simulink library "nmc"  (R2015b)
settings: Solver=ode45  SolverMode=SingleTasking  StartTime=0.0  StopTime=10.0  RelTol=1e-3
undefined symbols (not defined in the file): AnkleStance, AnkleSwing, c, c_jointstop, CtrlPar_FP_List, CtrlPar_FP_R_List, CtrlPar_LL_List, CtrlPar_St_List, CtrlPar_St_R_List, CtrlPar_Sw_List, CtrlPar_Sw_R_List, CtrlPar_theta0_List, CtrlPar_Tr_List, CtrlPar_Tr_R_List, CtrlPar_VelocityFile_List, D1G_HAT, eref, FmaxBFSH, FmaxGAS, FmaxGLU, FmaxHAB, FmaxHAD, FmaxHAM, FmaxHFL, FmaxRF, FmaxSOL, FmaxTA, FmaxVAS, init_a_tgt, init_a_tgtR, K, leg_l, LongDelay, LongLoopDelay, loptBFSH, loptGAS, loptGLU, loptHAB, loptHAD, loptHAM, loptHFL, loptRF, loptSOL, loptTA, loptVAS, lslackBFSH, lslackGAS, lslackGLU, lslackHAB, lslackHAD, lslackHAM, lslackHFL, lslackRF, lslackSOL, lslackTA, lslackVAS, magnitude, maxLoad_control_List, MeanStepsAnkle, MidDelay ... (+99)
libraries: nmc x63, simulink x31, simulink_extras x30, LopesDevelopmentLibrary x3
(part 3 of 10)

== system nmc/LopesToGeyer_angles/AnklePredictorRight/LeftSwing ==
  MeasPhase : Inport
  Clock : Clock
      settings: Decimation=1E6
  Constant : Constant  Value=MeanStepsAnkle
  "Frequency " : Stateflow chart  TreatAsAtomicUnit=on
  "mean_freq " : Outport
  count : Outport  Port=2
  wires:
  "Frequency "/1(count) -> count/1
  "Frequency "/2(mean_freq) -> "mean_freq "/1
  Clock/1 -> "Frequency "/1(time_sig)
  MeasPhase/1 -> "Frequency "/2(InSig)
  Constant/1 -> "Frequency "/3(N)

== system nmc/LopesToGeyer_angles/AnklePredictorRight/MeanReady? ==
  Compare To Constant : simulink/Logic and Bit Operations/Compare To Constant  relop=>  const=MeanStepsAnkle  OutDataTypeStr=boolean
  Compare To Constant1 : simulink/Logic and Bit Operations/Compare To Constant  relop=>  const=MeanStepsAnkle  OutDataTypeStr=boolean
  Logical Operator : Logic  AllPortsSameDT=off  OutDataTypeStr=boolean
  "Ready " : Outport
  wires:
  [CountStanceR] -> Compare To Constant/1
  [CountSwingR] -> Compare To Constant1/1
  Logical Operator/1 -> "Ready "/1
  Compare To Constant1/1 -> Logical Operator/1
  Compare To Constant/1 -> Logical Operator/2

== system nmc/LopesToGeyer_angles/AnklePredictorRight/Shape estimator left ==
  Cur_phase : Inport
  mean_freq_swing : Inport  Port=2
  mean_freq_stance : Inport  Port=3
  Enable : EnablePort  StatesWhenEnabling=reset  ZeroCross=off
  Compare To Constant : simulink/Logic and Bit Operations/Compare To Constant  relop===  const=0  OutDataTypeStr=boolean
  Compare To Constant1 : simulink/Logic and Bit Operations/Compare To Constant  relop===  const=1  OutDataTypeStr=boolean
  Cur_phase1 : InportShadow
  Phase 1 : Subsystem
  Phase 2 : Subsystem
  Switch : Switch  Criteria=u2 ~= 0
  Shape : Outport  OutputWhenDisabled=reset  InitialOutput=0
  wires:
  mean_freq_stance/1 -> Phase 2/1(mean_freq)
  mean_freq_swing/1 -> Phase 1/1(mean_freq)
  Compare To Constant1/1 -> Phase 2/Enable
  Compare To Constant/1 -> Phase 1/Enable
  Cur_phase1/1 -> Switch/2
  Phase 1/1(Shape_output) -> Switch/3
  Phase 2/1(Shape_output) -> Switch/1
  Switch/1 -> Shape/1
  Cur_phase/1 -> Compare To Constant1/1, Compare To Constant/1

== system nmc/NMC Model/Global to Body frame/body pitch//roll//yaw in body frame --- x-axis: forward y-axis: leftward z-axis: parallel to gravity ==
  LHip : Inport
  dLHip : Inport  Port=2
  HAT : Inport  Port=3
  dHAT : Inport  Port=4
  RHip : Inport  Port=5
  dRHip : Inport  Port=6
  " Mean Hip Speed" : Gain  Gain=1/2
  "Dx, Dy" : Selector  InputPortWidth=3  IndexOptions=Index vector (dialog)  Indices=[1 2]  OutputSizes=1
  "Dx, Dz" : Selector  InputPortWidth=3  IndexOptions=Index vector (dialog)  Indices=[1 3]  OutputSizes=1
  "Dx, Dz1" : Selector  InputPortWidth=3  IndexOptions=Index vector (dialog)  Indices=[1 3]  OutputSizes=1
  "Dz, Dy" : Selector  InputPortWidth=3  IndexOptions=Index vector (dialog)  Indices=[3 2]  OutputSizes=1
  Mean Hip Position : Gain  Gain=1/2
  Mux1 : Mux  Inputs=2
  Mux2 : Mux  Inputs=2
  Mux3 : Mux  Inputs=2
  Sum1 : Sum
  Sum2 : Sum
  Sum4 : Sum  Inputs=-+
  Sum5 : Sum  Inputs=+-
  Theta : Fcn  Expr=atan2(u(1),u(2))
  Theta1 : Fcn  Expr=atan2(u(1),u(2))
  "dDx, dDy" : Selector  InputPortWidth=3  IndexOptions=Index vector (dialog)  Indices=[1 2]  OutputSizes=1
  "dDz, dDy" : Selector  InputPortWidth=3  IndexOptions=Index vector (dialog)  Indices=[3 2]  OutputSizes=1
  dTheta : Fcn  Expr=( u(2)*u(3) - u(1)*u(4) ) / D1G_HAT^2
  dTheta1 : Fcn  Expr=( u(2)*u(3) - u(1)*u(4) ) / D1G_HAT^2
  map1 : Subsystem
  map2 : Subsystem
  new_bases : Subsystem
  yaw1 : Fcn  Expr=atan2(-u(1)+u(3),-u(2)+u(4))
  th_pitch : Outport
  dth_pitch : Outport  Port=2
  th_roll : Outport  Port=3
  dth_roll : Outport  Port=4
  yaw : Outport  Port=5
  wires:
  yaw1/1 -> yaw/1
  Mux3/1 -> yaw1/1
  "Dx, Dz1"/1 -> Mux3/2
  "Dx, Dz"/1 -> Mux3/1
  dTheta1/1 -> dth_roll/1
  Theta1/1 -> th_roll/1
  "Dz, Dy"/1 -> Theta1/1, Mux1/1
  Mux1/1 -> dTheta1/1
  "dDz, dDy"/1 -> Mux1/2
  map2/1(v_new) -> "dDz, dDy"/1, "dDx, dDy"/1
  Sum5/1 -> map2/1(v)
  new_bases/1(bases) -> map2/2(basis), map1/2(basis)
  map1/1(v_new) -> "Dz, Dy"/1, "Dx, Dy"/1
  Sum4/1 -> map1/1(v)
  dTheta/1 -> dth_pitch/1
  Theta/1 -> th_pitch/1
  dRHip/1 -> Sum2/2
  dLHip/1 -> Sum2/1
  RHip/1 -> "Dx, Dz1"/1, new_bases/2(R), Sum1/2
  LHip/1 -> "Dx, Dz"/1, new_bases/1(L), Sum1/1
  "Dx, Dy"/1 -> Theta/1, Mux2/1
  " Mean Hip Speed"/1 -> Sum5/2
  Mean Hip Position/1 -> Sum4/1
  HAT/1 -> Sum4/2
  Sum2/1 -> " Mean Hip Speed"/1
  Sum1/1 -> Mean Hip Position/1
  Mux2/1 -> dTheta/1
  "dDx, dDy"/1 -> Mux2/2
  dHAT/1 -> Sum5/1

== system nmc/NMC Model/Global to Body frame/lateral d, v in body frame (left) ==
  body yaw : Inport
  d0 : Inport  Port=2
  dist : Inport  Port=3
  vel : Inport  Port=4
  Mux1 : Mux  Inputs=2
  Mux2 : Mux  Inputs=2
  Mux3 : Mux  Inputs=2
  Sum : Sum  Inputs=-+|
  body frame in transverse plane (xz-plane)1 : Fcn  Expr=u(2)*sin(u(1)) + u(3)*cos(u(1))
  body frame in transverse plane (xz-plane)2 : Fcn  Expr=u(2)*sin(u(1)) + u(3)*cos(u(1))
  "d, v" : Outport
  wires:
  Mux3/1 -> "d, v"/1
  body frame in transverse plane (xz-plane)1/1 -> Mux3/1
  vel/1 -> Mux2/2
  body frame in transverse plane (xz-plane)2/1 -> Mux3/2
  dist/1 -> Sum/2
  d0/1 -> Sum/1
  Mux2/1 -> body frame in transverse plane (xz-plane)2/1
  body yaw/1 -> Mux1/1, Mux2/1
  Mux1/1 -> body frame in transverse plane (xz-plane)1/1
  Sum/1 -> Mux1/2

== system nmc/NMC Model/Global to Body frame/lateral d, v in body frame (right) ==
  body yaw : Inport
  d0 : Inport  Port=2
  dist : Inport  Port=3
  vel : Inport  Port=4
  Mux1 : Mux  Inputs=2
  Mux2 : Mux  Inputs=2
  Mux3 : Mux  Inputs=2
  Sum : Sum  Inputs=-+|
  body frame in transverse plane (xz-plane)1 : Fcn  Expr=u(2)*sin(u(1)) + u(3)*cos(u(1))
  body frame in transverse plane (xz-plane)2 : Fcn  Expr=u(2)*sin(u(1)) + u(3)*cos(u(1))
  "d, v" : Outport
  wires:
  Mux3/1 -> "d, v"/1
  body frame in transverse plane (xz-plane)1/1 -> Mux3/1
  vel/1 -> Mux2/2
  body frame in transverse plane (xz-plane)2/1 -> Mux3/2
  dist/1 -> Sum/2
  d0/1 -> Sum/1
  Mux2/1 -> body frame in transverse plane (xz-plane)2/1
  body yaw/1 -> Mux1/1, Mux2/1
  Mux1/1 -> body frame in transverse plane (xz-plane)1/1
  Sum/1 -> Mux1/2

== system nmc/NMC Model/Global to Body frame/sagittal d, v in body frame (left) ==
  body yaw : Inport
  d0 : Inport  Port=2
  dist : Inport  Port=3
  vel : Inport  Port=4
  Mux1 : Mux  Inputs=2
  Mux2 : Mux  Inputs=2
  Mux3 : Mux  Inputs=2
  Sum : Sum  Inputs=-+|
  body frame in transverse plane (xz-plane)1 : Fcn  Expr=u(2)*cos(u(1)) - u(3)*sin(u(1))
  body frame in transverse plane (xz-plane)2 : Fcn  Expr=u(2)*cos(u(1)) - u(3)*sin(u(1))
  "d, v" : Outport
  wires:
  Mux3/1 -> "d, v"/1
  body frame in transverse plane (xz-plane)1/1 -> Mux3/1
  vel/1 -> Mux2/2
  body frame in transverse plane (xz-plane)2/1 -> Mux3/2
  dist/1 -> Sum/2
  d0/1 -> Sum/1
  Mux2/1 -> body frame in transverse plane (xz-plane)2/1
  body yaw/1 -> Mux1/1, Mux2/1
  Mux1/1 -> body frame in transverse plane (xz-plane)1/1
  Sum/1 -> Mux1/2

== system nmc/NMC Model/Global to Body frame/sagittal d, v in body frame (right) ==
  body yaw : Inport
  d0 : Inport  Port=2
  dist : Inport  Port=3
  vel : Inport  Port=4
  Mux1 : Mux  Inputs=2
  Mux2 : Mux  Inputs=2
  Mux3 : Mux  Inputs=2
  Sum : Sum  Inputs=-+|
  body frame in transverse plane (xz-plane)1 : Fcn  Expr=u(2)*cos(u(1)) - u(3)*sin(u(1))
  body frame in transverse plane (xz-plane)2 : Fcn  Expr=u(2)*cos(u(1)) - u(3)*sin(u(1))
  "d, v" : Outport
  wires:
  Mux3/1 -> "d, v"/1
  body frame in transverse plane (xz-plane)1/1 -> Mux3/1
  vel/1 -> Mux2/2
  body frame in transverse plane (xz-plane)2/1 -> Mux3/2
  dist/1 -> Sum/2
  d0/1 -> Sum/1
  Mux2/1 -> body frame in transverse plane (xz-plane)2/1
  body yaw/1 -> Mux1/1, Mux2/1
  Mux1/1 -> body frame in transverse plane (xz-plane)1/1
  Sum/1 -> Mux1/2

== system nmc/NMC Model/Higher Control Layer (Supra Spinal Control)/Double Support ==
  LStance : Inport
  RStance : Inport  Port=2
  Lalpha_tgt : Inport  Port=3
  Lphi34 : Inport  Port=4
  Lphi23 : Inport  Port=5
  LHip_tgt : Inport  Port=6
  Lphi34R : Inport  Port=7
  Ralpha_tgt : Inport  Port=8
  Rphi34 : Inport  Port=9
  Rphi23 : Inport  Port=10
  RHip_tgt : Inport  Port=11
  Rphi34R : Inport  Port=12
  Abs{,1..3} (4 alike) : Abs  ZeroCross=off
  Lalpha' : Fcn  Expr=u(1) - u(2)/2
  Logical Operator1 : Logic  Operator=NOR  AllPortsSameDT=off  OutDataTypeStr=boolean
  Logical Operator2 : Logic  Operator=NOT  AllPortsSameDT=off
  Logical Operator3 : Logic  AllPortsSameDT=off
  Logical Operator4 : Logic  AllPortsSameDT=off
  Logical Operator5 : Logic  AllPortsSameDT=off
  Mux1 : Mux  Inputs=2
  Mux5 : Mux  Inputs=2
  Ralpha' : Fcn  Expr=u(1) - u(2)/2
  Relational Operator : RelationalOperator  Operator=>  ZeroCross=off
  Sum{1,3,5,7} (4 alike) : Sum  Inputs=-+|
  Sum2 : Sum  Inputs=++|
  Sum4 : Sum  Inputs=++|
  RonL : Outport
  Flight : Outport  Port=2
  LonR : Outport  Port=3
  wires:
  Logical Operator3/1 -> Logical Operator4/1, Logical Operator5/1
  Relational Operator/1 -> Logical Operator4/2, Logical Operator2/1
  Logical Operator5/1 -> LonR/1
  Logical Operator2/1 -> Logical Operator5/2
  Logical Operator4/1 -> RonL/1
  Sum4/1 -> Relational Operator/2
  Abs3/1 -> Sum4/1
  Abs/1 -> Sum4/2
  Sum3/1 -> Abs3/1
  Rphi34R/1 -> Sum3/2
  RHip_tgt/1 -> Sum3/1
  Sum2/1 -> Relational Operator/1
  Abs1/1 -> Sum2/2
  Abs2/1 -> Sum2/1
  Sum1/1 -> Abs2/1
  Lphi34R/1 -> Sum1/2
  LHip_tgt/1 -> Sum1/1
  Logical Operator1/1 -> Flight/1
  Rphi23/1 -> Mux1/2
  Rphi34/1 -> Mux1/1
  Ralpha_tgt/1 -> Sum5/1
  Lphi23/1 -> Mux5/2
  Lphi34/1 -> Mux5/1
  Lalpha_tgt/1 -> Sum7/1
  RStance/1 -> Logical Operator1/2, Logical Operator3/2
  LStance/1 -> Logical Operator1/1, Logical Operator3/1
  Sum7/1 -> Abs1/1
  Sum5/1 -> Abs/1
  Mux1/1 -> Ralpha'/1
  Ralpha'/1 -> Sum5/2
  Mux5/1 -> Lalpha'/1
  Lalpha'/1 -> Sum7/2  "Lalpha"

== system nmc/NMC Model/Higher Control Layer (Supra Spinal Control)/SpeedCheck ==
  Abs : Abs
  Abs1 : Abs
  Compare To Constant : simulink/Logic and Bit Operations/Compare To Constant  relop===  const=0  OutDataTypeStr=boolean
  Logical Operator : Logic  Operator=OR  Inputs=3  AllPortsSameDT=off  OutDataTypeStr=boolean
  Relational Operator : RelationalOperator  Operator=>  OutDataTypeStr=boolean
  Relational Operator1 : RelationalOperator  Operator=>  OutDataTypeStr=boolean
  Select_front_v : Selector  InputPortWidth=2  IndexOptions=Index vector (dialog)  Indices=[2]  OutputSizes=1
  Select_side_v : Selector  InputPortWidth=2  IndexOptions=Index vector (dialog)  Indices=[2]  OutputSizes=1
  StandingStill : Constant  Value=0
  Switch : Switch  Criteria=u2 > Threshold
  "Walking " : Constant
  WalkOrStop : Outport
  wires:
  Logical Operator/1 -> Switch/2
  [StandingStillLimitFront] -> Relational Operator/2
  StandingStill/1 -> Switch/3
  [EnableStandingStill] -> Compare To Constant/1
  Relational Operator1/1 -> Logical Operator/3
  Relational Operator/1 -> Logical Operator/2
  Switch/1 -> WalkOrStop/1
  Abs1/1 -> Relational Operator1/1
  Select_side_v/1 -> Abs1/1
  Compare To Constant/1 -> Logical Operator/1
  [side_dv_L] -> Select_side_v/1
  Abs/1 -> Relational Operator/1
  Select_front_v/1 -> Abs/1
  [front_dv_L] -> Select_front_v/1
  "Walking "/1 -> Switch/1
  [StandingStillLimitSide] -> Relational Operator1/2

== system nmc/NMC Model/Muscle Actuation Layer/L Ankle Joint Limits ==
  note: Ankle Joint Limits
  phi [rad] : Inport
  dphi [rad/s] : Inport  Port=2
  Gain1 : Gain  Gain=c_jointstop
  Gain2 : Gain  Gain=-1
  Gain3 : Gain  Gain=c_jointstop
  Gain4 : Gain  Gain=1/w_max_jointstop
  Mux1 : Mux  Inputs=2
  Mux3 : Mux  Inputs=2
  Overextension Torque : Fcn  Expr="- u(1)  *  (1-u(2)) * (u(2)<1) * (u(1)>0)"
  Overflexion Torque : Fcn  Expr="- u(1)  *  (1-u(2)) * (u(2)<1) * (u(1)<0)"
  Sum : Sum  Inputs=|+-
  Sum1 : Sum  Inputs=|+-
  Sum2 : Sum
  overextension angle : Constant  Value=phi12_UpLimit
  overflexion angle : Constant  Value=phi12_LowLimit
  M_stop [Nm] : Outport
  wires:
  Overextension Torque/1 -> Sum2/1
  Overflexion Torque/1 -> Sum2/2
  Gain2/1 -> Mux3/2
  Sum2/1 -> M_stop [Nm]/1
  Mux1/1 -> Overflexion Torque/1
  overflexion angle/1 -> Sum1/2
  Sum1/1 -> Gain1/1
  Gain1/1 -> Mux1/1
  Gain4/1 -> Mux1/2, Gain2/1
  Sum/1 -> Gain3/1
  phi [rad]/1 -> Sum1/1, Sum/1
  overextension angle/1 -> Sum/2
  dphi [rad/s]/1 -> Gain4/1
  Gain3/1 -> Mux3/1
  Mux3/1 -> Overextension Torque/1

== system nmc/NMC Model/Muscle Actuation Layer/L BFSH ==
  note: Excitation Contraction Coupling
  note: BFSH Muscle-Tendon Dynamics
  STIM : Inport
  lmtc [m] : Inport  Port=2
  1 : Product  Inputs=**  SaturateOnIntegerOverflow=on  InputSameDT=on  OutDataTypeStr=Inherit: Same as first input
  1/lslack : Gain  Gain=1/lslackBFSH  SaturateOnIntegerOverflow=on  OutDataTypeStr=Inherit: Same as input  ParamDataTypeStr=Inherit: Same as input
  BE force-length relation : Subsystem
  CE force-length relation : Subsystem
  CE inverse force-velocity relation : Subsystem
  Constant : Constant  Value=lslackBFSH
  ECC TransferFcn : simulink_extras/Additional Linear/Transfer Fcn (with initial outputs)  N=[1]  D="[tau  1]"  Y0=preA  U0=0
      settings: AttributesFormatString=pre-activation: %<Y0>
  Fmax : Gain  Gain=FmaxBFSH  SaturateOnIntegerOverflow=on  OutDataTypeStr=Inherit: Same as input  ParamDataTypeStr=Inherit: Same as input
  Fv = Fse / (A*Fce) : Product  Inputs=*/  SaturateOnIntegerOverflow=on  InputSameDT=on  OutDataTypeStr=Inherit: Same as first input
  Integrator : Integrator  InitialConditionSource=external  LowerSaturationLimit=0.05  ZeroCross=off
  PE force-length relation : Subsystem
  SE force-length relation : Subsystem
  Sum : Sum  Inputs=|+-  SaturateOnIntegerOverflow=on  InputSameDT=on  OutDataTypeStr=Inherit: Same as first input
  Sum2 : Sum  Inputs=|-+  SaturateOnIntegerOverflow=on  InputSameDT=on  OutDataTypeStr=Inherit: Same as first input
  Sum3 : Sum  SaturateOnIntegerOverflow=on  InputSameDT=on  OutDataTypeStr=Inherit: Same as first input
  Sum4 : Sum  SaturateOnIntegerOverflow=on  InputSameDT=on  OutDataTypeStr=Inherit: Same as first input
  lce/lopt : Gain  Gain=1/loptBFSH  SaturateOnIntegerOverflow=on  OutDataTypeStr=Inherit: Same as input  ParamDataTypeStr=Inherit: Same as input
  vmax*lopt : Gain  Gain=vmaxBFSH*loptBFSH  SaturateOnIntegerOverflow=on  OutDataTypeStr=Inherit: Same as input  ParamDataTypeStr=Inherit: Same as input
  Fmtc : Outport  InitialOutput=0
  Lce : Outport  Port=2  InitialOutput=0
  Vce : Outport  Port=3  InitialOutput=0
  A : Outport  Port=4  InitialOutput=0
  wires:
  ECC TransferFcn/1 -> 1/2, A/1
  STIM/1 -> ECC TransferFcn/1
  CE inverse force-velocity relation/1(v[vmax]) -> vmax*lopt/1
  Sum3/1 -> Fv = Fse / (A*Fce)/2
  BE force-length relation/1(fbe [Fmax]) -> Sum4/2
  1/1 -> Sum3/2
  PE force-length relation/1(fpe [Fmax]) -> Sum3/1
  Sum4/1 -> Fv = Fse / (A*Fce)/1
  CE force-length relation/1(fce [Fmax]) -> 1/1
  Constant/1 -> Sum2/1
  Sum2/1 -> Integrator/2
  SE force-length relation/1(fse [Fmax]) -> Sum4/1, Fmax/1
  1/lslack/1 -> SE force-length relation/1(lse [lslack])
  Fmax/1 -> Fmtc/1  "Fmtc"
  lmtc [m]/1 -> Sum/1, Sum2/2  "lmtc"
  vmax*lopt/1 -> Vce/1, Integrator/1  "vce"
  Fv = Fse / (A*Fce)/1 -> CE inverse force-velocity relation/1(Fv[Fmax])  "fv"
  lce/lopt/1 -> PE force-length relation/1(lce [lopt]), BE force-length relation/1(lce [lopt]), CE force-length relation/1(lce [lopt])
  Sum/1 -> 1/lslack/1  "lse"
  Integrator/1 -> Lce/1, lce/lopt/1, Sum/2  "lce"

== system nmc/NMC Model/Muscle Actuation Layer/L BFSH Link ==
  note: BFSH Attachment
  phi23 [rad] : Inport
  Constant : Constant  Value=lslackBFSH+loptBFSH
  Constant1 : Constant  Value=rBFSH
  Constant2 : Constant  Value=phirefBFSH
  Gain4 : Gain  Gain=rhoBFSH
  Product : Product  RndMeth=Zero
  Sum2 : Sum  Inputs=|+-
  Sum5 : Sum  Inputs=|++
  lmtu [m] : Outport
  lever [m] : Outport  Port=2
  wires:
  Constant1/1 -> lever [m]/1, Product/2
  Sum2/1 -> Product/1
  Constant2/1 -> Sum2/2
  phi23 [rad]/1 -> Sum2/1
  Product/1 -> Gain4/1
  Gain4/1 -> Sum5/2
  Sum5/1 -> lmtu [m]/1
  Constant/1 -> Sum5/1

== system nmc/NMC Model/Muscle Actuation Layer/L GAS ==
  note: Excitation Contraction Coupling
  note: GAS Muscle-Tendon Dynamics
  STIM : Inport
  lmtc [m] : Inport  Port=2
  1 : Product  Inputs=**  SaturateOnIntegerOverflow=on  InputSameDT=on  OutDataTypeStr=Inherit: Same as first input
  1/lslack : Gain  Gain=1/lslackGAS  SaturateOnIntegerOverflow=on  OutDataTypeStr=Inherit: Same as input  ParamDataTypeStr=Inherit: Same as input
  BE force-length relation : Subsystem
  CE force-length relation : Subsystem
  CE inverse force-velocity relation : Subsystem
  Constant : Constant  Value=lslackGAS
  ECC TransferFcn : simulink_extras/Additional Linear/Transfer Fcn (with initial outputs)  N=[1]  D="[tau  1]"  Y0=preA  U0=0
      settings: AttributesFormatString=pre-activation: %<Y0>
  Fmax : Gain  Gain=FmaxGAS  SaturateOnIntegerOverflow=on  OutDataTypeStr=Inherit: Same as input  ParamDataTypeStr=Inherit: Same as input
  Fv = Fse / (A*Fce) : Product  Inputs=*/  SaturateOnIntegerOverflow=on  InputSameDT=on  OutDataTypeStr=Inherit: Same as first input
  Integrator : Integrator  InitialConditionSource=external  LowerSaturationLimit=0.05  ZeroCross=off
  PE force-length relation : Subsystem
  SE force-length relation : Subsystem
  Sum : Sum  Inputs=|+-  SaturateOnIntegerOverflow=on  InputSameDT=on  OutDataTypeStr=Inherit: Same as first input
  Sum2 : Sum  Inputs=|-+  SaturateOnIntegerOverflow=on  InputSameDT=on  OutDataTypeStr=Inherit: Same as first input
  Sum3 : Sum  SaturateOnIntegerOverflow=on  InputSameDT=on  OutDataTypeStr=Inherit: Same as first input
  Sum4 : Sum  SaturateOnIntegerOverflow=on  InputSameDT=on  OutDataTypeStr=Inherit: Same as first input
  lce/lopt : Gain  Gain=1/loptGAS  SaturateOnIntegerOverflow=on  OutDataTypeStr=Inherit: Same as input  ParamDataTypeStr=Inherit: Same as input
  vmax*lopt : Gain  Gain=vmaxGAS*loptGAS  SaturateOnIntegerOverflow=on  OutDataTypeStr=Inherit: Same as input  ParamDataTypeStr=Inherit: Same as input
  Fmtc : Outport  InitialOutput=0
  Lce : Outport  Port=2  InitialOutput=0
  Vce : Outport  Port=3  InitialOutput=0
  A : Outport  Port=4  InitialOutput=0
  wires:
  ECC TransferFcn/1 -> 1/2, A/1
  STIM/1 -> ECC TransferFcn/1
  CE inverse force-velocity relation/1(v[vmax]) -> vmax*lopt/1
  Sum3/1 -> Fv = Fse / (A*Fce)/2
  BE force-length relation/1(fbe [Fmax]) -> Sum4/2
  1/1 -> Sum3/2
  PE force-length relation/1(fpe [Fmax]) -> Sum3/1
  Sum4/1 -> Fv = Fse / (A*Fce)/1
  CE force-length relation/1(fce [Fmax]) -> 1/1
  Constant/1 -> Sum2/1
  Sum2/1 -> Integrator/2
  SE force-length relation/1(fse [Fmax]) -> Sum4/1, Fmax/1
  1/lslack/1 -> SE force-length relation/1(lse [lslack])
  Fmax/1 -> Fmtc/1  "Fmtc"
  lmtc [m]/1 -> Sum/1, Sum2/2  "lmtc"
  vmax*lopt/1 -> Vce/1, Integrator/1  "vce"
  Fv = Fse / (A*Fce)/1 -> CE inverse force-velocity relation/1(Fv[Fmax])  "fv"
  lce/lopt/1 -> PE force-length relation/1(lce [lopt]), BE force-length relation/1(lce [lopt]), CE force-length relation/1(lce [lopt])
  Sum/1 -> 1/lslack/1  "lse"
  Integrator/1 -> Lce/1, lce/lopt/1, Sum/2  "lce"

== system nmc/NMC Model/Muscle Actuation Layer/L GAS Link ==
  note: GAS Attachment
  phi23 [rad] : Inport
  phi12 [rad] : Inport  Port=2
  Constant1 : Constant  Value=phimaxGASk
  Constant2 : Constant  Value=phirefGASk
  Constant3 : Constant  Value=phimaxGASa
  Constant4 : Constant  Value=lslackGAS+loptGAS
  Constant5 : Constant  Value=phirefGASa
  Demux : Demux  Outputs=2
  Demux1 : Demux  Outputs=2
  Gain1 : Gain  Gain=rGASkmax
  Gain2 : Gain  Gain=rGASamax
  Gain3 : Gain  Gain=phiScaleGASa
  Gain5 : Gain  Gain=phiScaleGASk
  Gain6 : Gain  Gain=phiScaleGASk
  Gain7 : Gain  Gain=rhoGASk/phiScaleGASk
  Gain8 : Gain  Gain=phiScaleGASa
  Gain9 : Gain  Gain=rhoGASa/phiScaleGASa
  Mux : Mux  Inputs=2
  Mux1 : Mux  Inputs=2
  Sum1 : Sum  Inputs=-+
  Sum2 : Sum  Inputs=|+-
  Sum3 : Sum  Inputs=-+|
  Sum4 : Sum  Inputs=-+
  Sum5 : Sum  Inputs=++-
  Sum6 : Sum  Inputs=|+-
  Sum7 : Sum  Inputs=-+|
  length change term : Trigonometry
  length change term1 : Trigonometry
  offset correction term : Trigonometry
  offset correction term1 : Trigonometry
  variable lever term : Trigonometry  Operator=cos
  variable lever term1 : Trigonometry  Operator=cos
  lmtu [m] : Outport
  lever23 [m] : Outport  Port=2
  lever12 [m] : Outport  Port=3
  wires:
  Gain8/1 -> offset correction term1/1
  Gain3/1 -> length change term1/1, variable lever term1/1
  Gain2/1 -> Demux1/1
  Mux1/1 -> Gain2/1
  variable lever term1/1 -> Mux1/2
  Sum4/1 -> Mux1/1
  offset correction term1/1 -> Sum4/1
  length change term1/1 -> Sum4/2
  Constant5/1 -> Sum6/1
  Sum6/1 -> Gain8/1
  Constant3/1 -> Sum6/2, Sum7/1
  Sum7/1 -> Gain3/1
  phi12 [rad]/1 -> Sum7/2
  Gain6/1 -> offset correction term/1
  Gain5/1 -> length change term/1, variable lever term/1
  Gain1/1 -> Demux/1
  Mux/1 -> Gain1/1
  variable lever term/1 -> Mux/2
  Sum1/1 -> Mux/1
  offset correction term/1 -> Sum1/1
  length change term/1 -> Sum1/2
  Constant2/1 -> Sum2/1
  Sum2/1 -> Gain6/1
  Constant1/1 -> Sum2/2, Sum3/1
  Sum3/1 -> Gain5/1
  phi23 [rad]/1 -> Sum3/2
  Gain7/1 -> Sum5/1
  Demux/1 -> Gain7/1
  Demux/2 -> lever23 [m]/1
  Gain9/1 -> Sum5/3
  Demux1/1 -> Gain9/1
  Constant4/1 -> Sum5/2
  Demux1/2 -> lever12 [m]/1
  Sum5/1 -> lmtu [m]/1

== system nmc/NMC Model/Muscle Actuation Layer/L GLU ==
  note: Excitation Contraction Coupling
  note: GLU Muscle-Tendon Dynamics
  STIM : Inport
  lmtc [m] : Inport  Port=2
  1 : Product  Inputs=**  SaturateOnIntegerOverflow=on  InputSameDT=on  OutDataTypeStr=Inherit: Same as first input
  1/lslack : Gain  Gain=1/lslackGLU  SaturateOnIntegerOverflow=on  OutDataTypeStr=Inherit: Same as input  ParamDataTypeStr=Inherit: Same as input
  BE force-length relation : Subsystem
  CE force-length relation : Subsystem
  CE inverse force-velocity relation : Subsystem
  Constant : Constant  Value=lslackGLU
  ECC TransferFcn : simulink_extras/Additional Linear/Transfer Fcn (with initial outputs)  N=[1]  D="[tau  1]"  Y0=preA  U0=0
      settings: AttributesFormatString=pre-activation: %<Y0>
  Fmax : Gain  Gain=FmaxGLU  SaturateOnIntegerOverflow=on  OutDataTypeStr=Inherit: Same as input  ParamDataTypeStr=Inherit: Same as input
  Fv = Fse / (A*Fce) : Product  Inputs=*/  SaturateOnIntegerOverflow=on  InputSameDT=on  OutDataTypeStr=Inherit: Same as first input
  Integrator : Integrator  InitialConditionSource=external  LowerSaturationLimit=0.05  ZeroCross=off
  PE force-length relation : Subsystem
  SE force-length relation : Subsystem
  Sum : Sum  Inputs=|+-  SaturateOnIntegerOverflow=on  InputSameDT=on  OutDataTypeStr=Inherit: Same as first input
  Sum2 : Sum  Inputs=|-+  SaturateOnIntegerOverflow=on  InputSameDT=on  OutDataTypeStr=Inherit: Same as first input
  Sum3 : Sum  SaturateOnIntegerOverflow=on  InputSameDT=on  OutDataTypeStr=Inherit: Same as first input
  Sum4 : Sum  SaturateOnIntegerOverflow=on  InputSameDT=on  OutDataTypeStr=Inherit: Same as first input
  lce/lopt : Gain  Gain=1/loptGLU  SaturateOnIntegerOverflow=on  OutDataTypeStr=Inherit: Same as input  ParamDataTypeStr=Inherit: Same as input
  vmax*lopt : Gain  Gain=vmaxGLU*loptGLU  SaturateOnIntegerOverflow=on  OutDataTypeStr=Inherit: Same as input  ParamDataTypeStr=Inherit: Same as input
  Fmtc : Outport  InitialOutput=0
  Lce : Outport  Port=2  InitialOutput=0
  Vce : Outport  Port=3  InitialOutput=0
  A : Outport  Port=4  InitialOutput=0
  wires:
  ECC TransferFcn/1 -> 1/2, A/1
  STIM/1 -> ECC TransferFcn/1
  CE inverse force-velocity relation/1(v[vmax]) -> vmax*lopt/1
  Sum3/1 -> Fv = Fse / (A*Fce)/2
  BE force-length relation/1(fbe [Fmax]) -> Sum4/2
  1/1 -> Sum3/2
  PE force-length relation/1(fpe [Fmax]) -> Sum3/1
  Sum4/1 -> Fv = Fse / (A*Fce)/1
  CE force-length relation/1(fce [Fmax]) -> 1/1
  Constant/1 -> Sum2/1
  Sum2/1 -> Integrator/2
  SE force-length relation/1(fse [Fmax]) -> Sum4/1, Fmax/1
  1/lslack/1 -> SE force-length relation/1(lse [lslack])
  Fmax/1 -> Fmtc/1  "Fmtc"
  lmtc [m]/1 -> Sum/1, Sum2/2  "lmtc"
  vmax*lopt/1 -> Vce/1, Integrator/1  "vce"
  Fv = Fse / (A*Fce)/1 -> CE inverse force-velocity relation/1(Fv[Fmax])  "fv"
  lce/lopt/1 -> PE force-length relation/1(lce [lopt]), BE force-length relation/1(lce [lopt]), CE force-length relation/1(lce [lopt])
  Sum/1 -> 1/lslack/1  "lse"
  Integrator/1 -> Lce/1, lce/lopt/1, Sum/2  "lce"

== system nmc/NMC Model/Muscle Actuation Layer/L GLU Link ==
  note: GLUTEUS Attachment
  phi34 [rad] : Inport
  Constant : Constant  Value=lslackGLU+loptGLU
  Constant1 : Constant  Value=rGLU
  Constant2 : Constant  Value=phirefGLU
  Gain2 : Gain  Gain=rhoGLU
  Product : Product  RndMeth=Zero
  Sum2 : Sum  Inputs=|+-
  Sum5 : Sum  Inputs=|+-
  lmtu [m] : Outport
  lever [m] : Outport  Port=2
  wires:
  Gain2/1 -> Sum5/2
  Constant1/1 -> lever [m]/1, Product/2
  Sum2/1 -> Product/1
  Constant2/1 -> Sum2/2
  phi34 [rad]/1 -> Sum2/1
  Product/1 -> Gain2/1
  Sum5/1 -> lmtu [m]/1
  Constant/1 -> Sum5/1

== system nmc/NMC Model/Muscle Actuation Layer/L HAB ==
  note: Excitation Contraction Coupling
  note: HAB Muscle-Tendon Dynamics
  STIM : Inport
  lmtc [m] : Inport  Port=2
  1 : Product  Inputs=**  SaturateOnIntegerOverflow=on  InputSameDT=on  OutDataTypeStr=Inherit: Same as first input
  1/lslack : Gain  Gain=1/lslackHAB  SaturateOnIntegerOverflow=on  OutDataTypeStr=Inherit: Same as input  ParamDataTypeStr=Inherit: Same as input
  BE force-length relation : Subsystem
  CE force-length relation : Subsystem
  CE inverse force-velocity relation : Subsystem
  Constant : Constant  Value=lslackHAB
  ECC TransferFcn : simulink_extras/Additional Linear/Transfer Fcn (with initial outputs)  N=[1]  D="[tau  1]"  Y0=preA  U0=0
      settings: AttributesFormatString=pre-activation: %<Y0>
  Fmax : Gain  Gain=FmaxHAB  SaturateOnIntegerOverflow=on  OutDataTypeStr=Inherit: Same as input  ParamDataTypeStr=Inherit: Same as input
  Fv = Fse / (A*Fce) : Product  Inputs=*/  SaturateOnIntegerOverflow=on  InputSameDT=on  OutDataTypeStr=Inherit: Same as first input
  Integrator : Integrator  InitialConditionSource=external  LowerSaturationLimit=0.05  ZeroCross=off
  PE force-length relation : Subsystem
  SE force-length relation : Subsystem
  Sum : Sum  Inputs=|+-  SaturateOnIntegerOverflow=on  InputSameDT=on  OutDataTypeStr=Inherit: Same as first input
  Sum2 : Sum  Inputs=|-+  SaturateOnIntegerOverflow=on  InputSameDT=on  OutDataTypeStr=Inherit: Same as first input
  Sum3 : Sum  SaturateOnIntegerOverflow=on  InputSameDT=on  OutDataTypeStr=Inherit: Same as first input
  Sum4 : Sum  SaturateOnIntegerOverflow=on  InputSameDT=on  OutDataTypeStr=Inherit: Same as first input
  lce/lopt : Gain  Gain=1/loptHAB  SaturateOnIntegerOverflow=on  OutDataTypeStr=Inherit: Same as input  ParamDataTypeStr=Inherit: Same as input
  vmax*lopt : Gain  Gain=vmaxHAB*loptHAB  SaturateOnIntegerOverflow=on  OutDataTypeStr=Inherit: Same as input  ParamDataTypeStr=Inherit: Same as input
  Fmtc : Outport  InitialOutput=0
  Lce : Outport  Port=2  InitialOutput=0
  Vce : Outport  Port=3  InitialOutput=0
  A : Outport  Port=4  InitialOutput=0
  wires:
  ECC TransferFcn/1 -> 1/2, A/1
  STIM/1 -> ECC TransferFcn/1
  CE inverse force-velocity relation/1(v[vmax]) -> vmax*lopt/1
  Sum3/1 -> Fv = Fse / (A*Fce)/2
  BE force-length relation/1(fbe [Fmax]) -> Sum4/2
  1/1 -> Sum3/2
  PE force-length relation/1(fpe [Fmax]) -> Sum3/1
  Sum4/1 -> Fv = Fse / (A*Fce)/1
  CE force-length relation/1(fce [Fmax]) -> 1/1
  Constant/1 -> Sum2/1
  Sum2/1 -> Integrator/2
  SE force-length relation/1(fse [Fmax]) -> Sum4/1, Fmax/1
  1/lslack/1 -> SE force-length relation/1(lse [lslack])
  Fmax/1 -> Fmtc/1  "Fmtc"
  lmtc [m]/1 -> Sum/1, Sum2/2  "lmtc"
  vmax*lopt/1 -> Vce/1, Integrator/1  "vce"
  Fv = Fse / (A*Fce)/1 -> CE inverse force-velocity relation/1(Fv[Fmax])  "fv"
  lce/lopt/1 -> PE force-length relation/1(lce [lopt]), BE force-length relation/1(lce [lopt]), CE force-length relation/1(lce [lopt])
  Sum/1 -> 1/lslack/1  "lse"
  Integrator/1 -> Lce/1, lce/lopt/1, Sum/2  "lce"

== system nmc/NMC Model/Muscle Actuation Layer/L HAB Link ==
  note: HAB Attachment
  phi34R [rad] : Inport
  Constant : Constant  Value=lslackHAB+loptHAB
  Constant1 : Constant  Value=rHAB
  Constant2 : Constant  Value=phirefHAB
  Gain2 : Gain  Gain=rhoHAB
  Product : Product  RndMeth=Zero
  Sum2 : Sum  Inputs=|+-
  Sum5 : Sum  Inputs=|+-
  lmtu [m] : Outport
  lever [m] : Outport  Port=2
  wires:
  Gain2/1 -> Sum5/2
  Constant1/1 -> lever [m]/1, Product/2
  Sum2/1 -> Product/1
  Constant2/1 -> Sum2/2
  phi34R [rad]/1 -> Sum2/1
  Product/1 -> Gain2/1
  Sum5/1 -> lmtu [m]/1
  Constant/1 -> Sum5/1

== system nmc/NMC Model/Muscle Actuation Layer/L HAD ==
  note: Excitation Contraction Coupling
  note: HAD Muscle-Tendon Dynamics
  STIM : Inport
  lmtc [m] : Inport  Port=2
  1 : Product  Inputs=**  SaturateOnIntegerOverflow=on  InputSameDT=on  OutDataTypeStr=Inherit: Same as first input
  1/lslack : Gain  Gain=1/lslackHAD  SaturateOnIntegerOverflow=on  OutDataTypeStr=Inherit: Same as input  ParamDataTypeStr=Inherit: Same as input
  BE force-length relation : Subsystem
  CE force-length relation : Subsystem
  CE inverse force-velocity relation : Subsystem
  Constant : Constant  Value=lslackHAD
  ECC TransferFcn : simulink_extras/Additional Linear/Transfer Fcn (with initial outputs)  N=[1]  D="[tau  1]"  Y0=preA  U0=0
      settings: AttributesFormatString=pre-activation: %<Y0>
  Fmax : Gain  Gain=FmaxHAD  SaturateOnIntegerOverflow=on  OutDataTypeStr=Inherit: Same as input  ParamDataTypeStr=Inherit: Same as input
  Fv = Fse / (A*Fce) : Product  Inputs=*/  SaturateOnIntegerOverflow=on  InputSameDT=on  OutDataTypeStr=Inherit: Same as first input
  Integrator : Integrator  InitialConditionSource=external  LowerSaturationLimit=0.05  ZeroCross=off
  PE force-length relation : Subsystem
  SE force-length relation : Subsystem
  Sum : Sum  Inputs=|+-  SaturateOnIntegerOverflow=on  InputSameDT=on  OutDataTypeStr=Inherit: Same as first input
  Sum2 : Sum  Inputs=|-+  SaturateOnIntegerOverflow=on  InputSameDT=on  OutDataTypeStr=Inherit: Same as first input
  Sum3 : Sum  SaturateOnIntegerOverflow=on  InputSameDT=on  OutDataTypeStr=Inherit: Same as first input
  Sum4 : Sum  SaturateOnIntegerOverflow=on  InputSameDT=on  OutDataTypeStr=Inherit: Same as first input
  lce/lopt : Gain  Gain=1/loptHAD  SaturateOnIntegerOverflow=on  OutDataTypeStr=Inherit: Same as input  ParamDataTypeStr=Inherit: Same as input
  vmax*lopt : Gain  Gain=vmaxHAD*loptHAD  SaturateOnIntegerOverflow=on  OutDataTypeStr=Inherit: Same as input  ParamDataTypeStr=Inherit: Same as input
  Fmtc : Outport  InitialOutput=0
  Lce : Outport  Port=2  InitialOutput=0
  Vce : Outport  Port=3  InitialOutput=0
  A : Outport  Port=4  InitialOutput=0
  wires:
  ECC TransferFcn/1 -> 1/2, A/1
  STIM/1 -> ECC TransferFcn/1
  CE inverse force-velocity relation/1(v[vmax]) -> vmax*lopt/1
  Sum3/1 -> Fv = Fse / (A*Fce)/2
  BE force-length relation/1(fbe [Fmax]) -> Sum4/2
  1/1 -> Sum3/2
  PE force-length relation/1(fpe [Fmax]) -> Sum3/1
  Sum4/1 -> Fv = Fse / (A*Fce)/1
  CE force-length relation/1(fce [Fmax]) -> 1/1
  Constant/1 -> Sum2/1
  Sum2/1 -> Integrator/2
  SE force-length relation/1(fse [Fmax]) -> Sum4/1, Fmax/1
  1/lslack/1 -> SE force-length relation/1(lse [lslack])
  Fmax/1 -> Fmtc/1  "Fmtc"
  lmtc [m]/1 -> Sum/1, Sum2/2  "lmtc"
  vmax*lopt/1 -> Vce/1, Integrator/1  "vce"
  Fv = Fse / (A*Fce)/1 -> CE inverse force-velocity relation/1(Fv[Fmax])  "fv"
  lce/lopt/1 -> PE force-length relation/1(lce [lopt]), BE force-length relation/1(lce [lopt]), CE force-length relation/1(lce [lopt])
  Sum/1 -> 1/lslack/1  "lse"
  Integrator/1 -> Lce/1, lce/lopt/1, Sum/2  "lce"

== system nmc/NMC Model/Muscle Actuation Layer/L HAD Link ==
  note: HAD Attachment
  phi34R [rad] : Inport
  Constant : Constant  Value=lslackHAD+loptHAD
  Constant1 : Constant  Value=rHAD
  Constant2 : Constant  Value=phirefHAD
  Gain2 : Gain  Gain=rhoHAD
  Product : Product  RndMeth=Zero
  Sum2 : Sum  Inputs=|+-
  Sum5 : Sum  Inputs=|++
  lmtu [m] : Outport
  lever [m] : Outport  Port=2
  wires:
  Gain2/1 -> Sum5/2
  Constant1/1 -> lever [m]/1, Product/2
  Sum2/1 -> Product/1
  Constant2/1 -> Sum2/2
  phi34R [rad]/1 -> Sum2/1
  Product/1 -> Gain2/1
  Sum5/1 -> lmtu [m]/1
  Constant/1 -> Sum5/1

== system nmc/NMC Model/Muscle Actuation Layer/L HAM ==
  note: Excitation Contraction Coupling
  note: HAM Muscle-Tendon Dynamics
  STIM : Inport
  lmtc [m] : Inport  Port=2
  1 : Product  Inputs=**  SaturateOnIntegerOverflow=on  InputSameDT=on  OutDataTypeStr=Inherit: Same as first input
  1/lslack : Gain  Gain=1/lslackHAM  SaturateOnIntegerOverflow=on  OutDataTypeStr=Inherit: Same as input  ParamDataTypeStr=Inherit: Same as input
  BE force-length relation : Subsystem
  CE force-length relation : Subsystem
  CE inverse force-velocity relation : Subsystem
  Constant : Constant  Value=lslackHAM
  ECC TransferFcn : simulink_extras/Additional Linear/Transfer Fcn (with initial outputs)  N=[1]  D="[tau  1]"  Y0=preA  U0=0
      settings: AttributesFormatString=pre-activation: %<Y0>
  Fmax : Gain  Gain=FmaxHAM  SaturateOnIntegerOverflow=on  OutDataTypeStr=Inherit: Same as input  ParamDataTypeStr=Inherit: Same as input
  Fv = Fse / (A*Fce) : Product  Inputs=*/  SaturateOnIntegerOverflow=on  InputSameDT=on  OutDataTypeStr=Inherit: Same as first input
  Integrator : Integrator  InitialConditionSource=external  LowerSaturationLimit=0.05  ZeroCross=off
  PE force-length relation : Subsystem
  SE force-length relation : Subsystem
  Sum : Sum  Inputs=|+-  SaturateOnIntegerOverflow=on  InputSameDT=on  OutDataTypeStr=Inherit: Same as first input
  Sum2 : Sum  Inputs=|-+  SaturateOnIntegerOverflow=on  InputSameDT=on  OutDataTypeStr=Inherit: Same as first input
  Sum3 : Sum  SaturateOnIntegerOverflow=on  InputSameDT=on  OutDataTypeStr=Inherit: Same as first input
  Sum4 : Sum  SaturateOnIntegerOverflow=on  InputSameDT=on  OutDataTypeStr=Inherit: Same as first input
  lce/lopt : Gain  Gain=1/loptHAM  SaturateOnIntegerOverflow=on  OutDataTypeStr=Inherit: Same as input  ParamDataTypeStr=Inherit: Same as input
  vmax*lopt : Gain  Gain=vmaxHAM*loptHAM  SaturateOnIntegerOverflow=on  OutDataTypeStr=Inherit: Same as input  ParamDataTypeStr=Inherit: Same as input
  Fmtc : Outport  InitialOutput=0
  Lce : Outport  Port=2  InitialOutput=0
  Vce : Outport  Port=3  InitialOutput=0
  A : Outport  Port=4  InitialOutput=0
  wires:
  ECC TransferFcn/1 -> A/1, 1/2
  STIM/1 -> ECC TransferFcn/1
  CE inverse force-velocity relation/1(v[vmax]) -> vmax*lopt/1
  Sum3/1 -> Fv = Fse / (A*Fce)/2
  BE force-length relation/1(fbe [Fmax]) -> Sum4/2
  1/1 -> Sum3/2
  PE force-length relation/1(fpe [Fmax]) -> Sum3/1
  Sum4/1 -> Fv = Fse / (A*Fce)/1
  CE force-length relation/1(fce [Fmax]) -> 1/1
  Constant/1 -> Sum2/1
  Sum2/1 -> Integrator/2
  SE force-length relation/1(fse [Fmax]) -> Sum4/1, Fmax/1
  1/lslack/1 -> SE force-length relation/1(lse [lslack])
  Fmax/1 -> Fmtc/1  "Fmtc"
  lmtc [m]/1 -> Sum/1, Sum2/2  "lmtc"
  vmax*lopt/1 -> Vce/1, Integrator/1  "vce"
  Fv = Fse / (A*Fce)/1 -> CE inverse force-velocity relation/1(Fv[Fmax])  "fv"
  lce/lopt/1 -> PE force-length relation/1(lce [lopt]), BE force-length relation/1(lce [lopt]), CE force-length relation/1(lce [lopt])
  Sum/1 -> 1/lslack/1  "lse"
  Integrator/1 -> Lce/1, lce/lopt/1, Sum/2  "lce"

== system nmc/NMC Model/Muscle Actuation Layer/L HAM Link ==
  note: HAM Attachment
  phi34 [rad] : Inport
  phi23 [rad] : Inport  Port=2
  Constant1 : Constant  Value=rHAMk
  Constant2 : Constant  Value=phirefHAMk
  Constant3 : Constant  Value=rHAMh
  Constant4 : Constant  Value=lslackHAM+loptHAM
  Constant5 : Constant  Value=phirefHAMh
  Gain2 : Gain  Gain=rhoHAMh
  Gain4 : Gain  Gain=rhoHAMk
  Product : Product  RndMeth=Zero
  Product1 : Product  RndMeth=Zero
  Sum1 : Sum  Inputs=|+-
  Sum4 : Sum  Inputs=|+-
  Sum5 : Sum  Inputs=-++
  lmtu [m] : Outport
  lever34 [m] : Outport  Port=2
  lever23 [m] : Outport  Port=3
  wires:
  Product1/1 -> Gain4/1
  Constant1/1 -> lever23 [m]/1, Product1/2
  Sum1/1 -> Product1/1
  Constant2/1 -> Sum1/2
  phi23 [rad]/1 -> Sum1/1
  Product/1 -> Gain2/1
  Constant3/1 -> lever34 [m]/1, Product/2
  Sum4/1 -> Product/1
  Constant5/1 -> Sum4/2
  phi34 [rad]/1 -> Sum4/1
  Gain2/1 -> Sum5/1
  Gain4/1 -> Sum5/3
  Constant4/1 -> Sum5/2
  Sum5/1 -> lmtu [m]/1

== system nmc/NMC Model/Muscle Actuation Layer/L HFL ==
  note: HFL Muscle-Tendon Dynamics
  STIM : Inport
  lmtc [m] : Inport  Port=2
  1 : Product  Inputs=**  SaturateOnIntegerOverflow=on  InputSameDT=on  OutDataTypeStr=Inherit: Same as first input
  1/lslack : Gain  Gain=1/lslackHFL  SaturateOnIntegerOverflow=on  OutDataTypeStr=Inherit: Same as input  ParamDataTypeStr=Inherit: Same as input
  BE force-length relation : Subsystem
  CE force-length relation : Subsystem
  CE inverse force-velocity relation : Subsystem
  Constant : Constant  Value=lslackHFL
  ECC TransferFcn : simulink_extras/Additional Linear/Transfer Fcn (with initial outputs)  N=[1]  D="[tau  1]"  Y0=preA  U0=0
      settings: AttributesFormatString=pre-activation: %<Y0>
  Fmax : Gain  Gain=FmaxHFL  SaturateOnIntegerOverflow=on  OutDataTypeStr=Inherit: Same as input  ParamDataTypeStr=Inherit: Same as input
  Fv = Fse / (A*Fce) : Product  Inputs=*/  SaturateOnIntegerOverflow=on  InputSameDT=on  OutDataTypeStr=Inherit: Same as first input
  Integrator : Integrator  InitialConditionSource=external  LowerSaturationLimit=0.05  ZeroCross=off
  PE force-length relation : Subsystem
  SE force-length relation : Subsystem
  Sum : Sum  Inputs=|+-  SaturateOnIntegerOverflow=on  InputSameDT=on  OutDataTypeStr=Inherit: Same as first input
  Sum2 : Sum  Inputs=|-+  SaturateOnIntegerOverflow=on  InputSameDT=on  OutDataTypeStr=Inherit: Same as first input
  Sum3 : Sum  SaturateOnIntegerOverflow=on  InputSameDT=on  OutDataTypeStr=Inherit: Same as first input
  Sum4 : Sum  SaturateOnIntegerOverflow=on  InputSameDT=on  OutDataTypeStr=Inherit: Same as first input
  lce/lopt : Gain  Gain=1/loptHFL  SaturateOnIntegerOverflow=on  OutDataTypeStr=Inherit: Same as input  ParamDataTypeStr=Inherit: Same as input
  vmax*lopt : Gain  Gain=vmaxHFL*loptHFL  SaturateOnIntegerOverflow=on  OutDataTypeStr=Inherit: Same as input  ParamDataTypeStr=Inherit: Same as input
  Fmtc : Outport  InitialOutput=0
  Lce : Outport  Port=2  InitialOutput=0
  Vce : Outport  Port=3  InitialOutput=0
  A : Outport  Port=4  InitialOutput=0
  wires:
  CE inverse force-velocity relation/1(v[vmax]) -> vmax*lopt/1
  ECC TransferFcn/1 -> 1/2, A/1
  STIM/1 -> ECC TransferFcn/1
  Sum3/1 -> Fv = Fse / (A*Fce)/2
  BE force-length relation/1(fbe [Fmax]) -> Sum4/2
  1/1 -> Sum3/2
  PE force-length relation/1(fpe [Fmax]) -> Sum3/1
  Sum4/1 -> Fv = Fse / (A*Fce)/1
  CE force-length relation/1(fce [Fmax]) -> 1/1
  Constant/1 -> Sum2/1
  Sum2/1 -> Integrator/2
  SE force-length relation/1(fse [Fmax]) -> Sum4/1, Fmax/1
  1/lslack/1 -> SE force-length relation/1(lse [lslack])
  Fmax/1 -> Fmtc/1  "Fmtc"
  lmtc [m]/1 -> Sum/1, Sum2/2  "lmtc"
  vmax*lopt/1 -> Vce/1, Integrator/1  "vce"
  Fv = Fse / (A*Fce)/1 -> CE inverse force-velocity relation/1(Fv[Fmax])  "fv"
  lce/lopt/1 -> PE force-length relation/1(lce [lopt]), BE force-length relation/1(lce [lopt]), CE force-length relation/1(lce [lopt])
  Sum/1 -> 1/lslack/1  "lse"
  Integrator/1 -> Lce/1, lce/lopt/1, Sum/2  "lce"

== system nmc/NMC Model/Muscle Actuation Layer/L HFL Link ==
  note: HFL Attachment
  phi34 [rad] : Inport
  Constant : Constant  Value=lslackHFL+loptHFL
  Constant1 : Constant  Value=rHFL
  Constant2 : Constant  Value=phirefHFL
  Gain2 : Gain  Gain=rhoHFL
  Product : Product  RndMeth=Zero
  Sum2 : Sum  Inputs=|+-
  Sum5 : Sum  Inputs=|++
  lmtu [m] : Outport
  lever [m] : Outport  Port=2
  wires:
  Constant1/1 -> lever [m]/1, Product/2
  Gain2/1 -> Sum5/2
  Sum2/1 -> Product/1
  Constant2/1 -> Sum2/2
  phi34 [rad]/1 -> Sum2/1
  Product/1 -> Gain2/1
  Sum5/1 -> lmtu [m]/1
  Constant/1 -> Sum5/1

== system nmc/NMC Model/Muscle Actuation Layer/L Hip Joint Limits ==
  note: Ankle Joint Limits
  phi [rad] : Inport
  dphi [rad/s] : Inport  Port=2
  Gain2 : Gain  Gain=-1
  Gain3 : Gain  Gain=c_jointstop
  Gain4 : Gain  Gain=1/w_max_jointstop
  Mux3 : Mux  Inputs=2
  Overextension Torque : Fcn  Expr="- u(1)  *  (1-u(2)) * (u(2)<1) * (u(1)>0)"
  Sum : Sum  Inputs=|+-
  overextension angle : Constant  Value=phi34_UpLimit
  M_stop [Nm] : Outport
  wires:
  Overextension Torque/1 -> M_stop [Nm]/1
  Gain2/1 -> Mux3/2
  Gain4/1 -> Gain2/1
  Sum/1 -> Gain3/1
  phi [rad]/1 -> Sum/1
  overextension angle/1 -> Sum/2
  dphi [rad/s]/1 -> Gain4/1
  Gain3/1 -> Mux3/1
  Mux3/1 -> Overextension Torque/1

== system nmc/NMC Model/Muscle Actuation Layer/L Hip Roll Joint Limits ==
  note: Ankle Joint Limits
  phi [rad] : Inport
  dphi [rad/s] : Inport  Port=2
  Gain1 : Gain  Gain=c_jointstop
  Gain2 : Gain  Gain=-1
  Gain3 : Gain  Gain=c_jointstop
  Gain4 : Gain  Gain=1/w_max_jointstop
  Mux1 : Mux  Inputs=2
  Mux3 : Mux  Inputs=2
  Overextension Torque : Fcn  Expr="- u(1)  *  (1-u(2)) * (u(2)<1) * (u(1)>0)"
  Overflexion Torque : Fcn  Expr="- u(1)  *  (1-u(2)) * (u(2)<1) * (u(1)<0)"
  Sum : Sum  Inputs=|+-
  Sum1 : Sum  Inputs=|+-
  Sum2 : Sum
  overextension angle : Constant  Value=phi34R_UpLimit
  overflexion angle : Constant  Value=phi34R_LowLimit
  M_stop [Nm] : Outport
  wires:
  Overextension Torque/1 -> Sum2/1
  Overflexion Torque/1 -> Sum2/2
  Gain2/1 -> Mux3/2
  Sum2/1 -> M_stop [Nm]/1
  Mux1/1 -> Overflexion Torque/1
  overflexion angle/1 -> Sum1/2
  Sum1/1 -> Gain1/1
  Gain1/1 -> Mux1/1
  Gain4/1 -> Mux1/2, Gain2/1
  Sum/1 -> Gain3/1
  phi [rad]/1 -> Sum1/1, Sum/1
  overextension angle/1 -> Sum/2
  dphi [rad/s]/1 -> Gain4/1
  Gain3/1 -> Mux3/1
  Mux3/1 -> Overextension Torque/1

== system nmc/NMC Model/Muscle Actuation Layer/L Knee Joint Limits ==
  note: Ankle Joint Limits
  phi [rad] : Inport
  dphi [rad/s] : Inport  Port=2
  Gain2 : Gain  Gain=-1
  Gain3 : Gain  Gain=c_jointstop
  Gain4 : Gain  Gain=1/w_max_jointstop
  Mux3 : Mux  Inputs=2
  Overextension Torque : Fcn  Expr="- u(1)  *  (1-u(2)) * (u(2)<1) * (u(1)>0)"
  Sum : Sum  Inputs=|+-
  overextension angle : Constant  Value=phi23_UpLimit
  M_stop [Nm] : Outport
  wires:
  Overextension Torque/1 -> M_stop [Nm]/1
  Gain2/1 -> Mux3/2
  Gain4/1 -> Gain2/1
  Sum/1 -> Gain3/1
  phi [rad]/1 -> Sum/1
  overextension angle/1 -> Sum/2
  dphi [rad/s]/1 -> Gain4/1
  Gain3/1 -> Mux3/1
  Mux3/1 -> Overextension Torque/1

== system nmc/NMC Model/Muscle Actuation Layer/L RF ==
  note: Excitation Contraction Coupling
  note: RF Muscle-Tendon Dynamics
  STIM : Inport
  lmtc [m] : Inport  Port=2
  1 : Product  Inputs=**  SaturateOnIntegerOverflow=on  InputSameDT=on  OutDataTypeStr=Inherit: Same as first input
  1/lslack : Gain  Gain=1/lslackRF  SaturateOnIntegerOverflow=on  OutDataTypeStr=Inherit: Same as input  ParamDataTypeStr=Inherit: Same as input
  BE force-length relation : Subsystem
  CE force-length relation : Subsystem
  CE inverse force-velocity relation : Subsystem
  Constant : Constant  Value=lslackRF
  ECC TransferFcn : simulink_extras/Additional Linear/Transfer Fcn (with initial outputs)  N=[1]  D="[tau  1]"  Y0=preA  U0=0
      settings: AttributesFormatString=pre-activation: %<Y0>
  Fmax : Gain  Gain=FmaxRF  SaturateOnIntegerOverflow=on  OutDataTypeStr=Inherit: Same as input  ParamDataTypeStr=Inherit: Same as input
  Fv = Fse / (A*Fce) : Product  Inputs=*/  SaturateOnIntegerOverflow=on  InputSameDT=on  OutDataTypeStr=Inherit: Same as first input
  Integrator : Integrator  InitialConditionSource=external  LowerSaturationLimit=0.05  ZeroCross=off
  PE force-length relation : Subsystem
  SE force-length relation : Subsystem
  Sum : Sum  Inputs=|+-  SaturateOnIntegerOverflow=on  InputSameDT=on  OutDataTypeStr=Inherit: Same as first input
  Sum2 : Sum  Inputs=|-+  SaturateOnIntegerOverflow=on  InputSameDT=on  OutDataTypeStr=Inherit: Same as first input
  Sum3 : Sum  SaturateOnIntegerOverflow=on  InputSameDT=on  OutDataTypeStr=Inherit: Same as first input
  Sum4 : Sum  SaturateOnIntegerOverflow=on  InputSameDT=on  OutDataTypeStr=Inherit: Same as first input
  lce/lopt : Gain  Gain=1/loptRF  SaturateOnIntegerOverflow=on  OutDataTypeStr=Inherit: Same as input  ParamDataTypeStr=Inherit: Same as input
  vmax*lopt : Gain  Gain=vmaxRF*loptRF  SaturateOnIntegerOverflow=on  OutDataTypeStr=Inherit: Same as input  ParamDataTypeStr=Inherit: Same as input
  Fmtc : Outport  InitialOutput=0
  Lce : Outport  Port=2  InitialOutput=0
  Vce : Outport  Port=3  InitialOutput=0
  A : Outport  Port=4  InitialOutput=0
  wires:
  ECC TransferFcn/1 -> A/1, 1/2
  STIM/1 -> ECC TransferFcn/1
  CE inverse force-velocity relation/1(v[vmax]) -> vmax*lopt/1
  Sum3/1 -> Fv = Fse / (A*Fce)/2
  BE force-length relation/1(fbe [Fmax]) -> Sum4/2
  1/1 -> Sum3/2
  PE force-length relation/1(fpe [Fmax]) -> Sum3/1
  Sum4/1 -> Fv = Fse / (A*Fce)/1
  CE force-length relation/1(fce [Fmax]) -> 1/1
  Constant/1 -> Sum2/1
  Sum2/1 -> Integrator/2
  SE force-length relation/1(fse [Fmax]) -> Sum4/1, Fmax/1
  1/lslack/1 -> SE force-length relation/1(lse [lslack])
  Fmax/1 -> Fmtc/1  "Fmtc"
  lmtc [m]/1 -> Sum/1, Sum2/2  "lmtc"
  vmax*lopt/1 -> Vce/1, Integrator/1  "vce"
  Fv = Fse / (A*Fce)/1 -> CE inverse force-velocity relation/1(Fv[Fmax])  "fv"
  lce/lopt/1 -> PE force-length relation/1(lce [lopt]), BE force-length relation/1(lce [lopt]), CE force-length relation/1(lce [lopt])
  Sum/1 -> 1/lslack/1  "lse"
  Integrator/1 -> Lce/1, lce/lopt/1, Sum/2  "lce"

== system nmc/NMC Model/Muscle Actuation Layer/L RF Link ==
  note: RF Attachment
  phi34 [rad] : Inport
  phi23 [rad] : Inport  Port=2
  Constant1 : Constant  Value=phimaxRFk
  Constant2 : Constant  Value=phirefRFk
  Constant3 : Constant  Value=rRFh
  Constant4 : Constant  Value=lslackRF+loptRF
  Constant5 : Constant  Value=phirefRFh
  Demux : Demux  Outputs=2
  Gain1 : Gain  Gain=rRFkmax
  Gain2 : Gain  Gain=rhoRFh
  Gain3 : Gain  Gain=phiScaleRFk
  Gain4 : Gain  Gain=rhoRFk/phiScaleRFk
  Gain5 : Gain  Gain=phiScaleRFk
  Mux : Mux  Inputs=2
  Product : Product  RndMeth=Zero
  Sum1 : Sum  Inputs=-+
  Sum2 : Sum  Inputs=|+-
  Sum3 : Sum  Inputs=-+|
  Sum4 : Sum  Inputs=|+-
  Sum5 : Sum  Inputs=++-
  length change term : Trigonometry
  offset correction term : Trigonometry
  variable lever term : Trigonometry  Operator=cos
  lmtu [m] : Outport
  lever34 [m] : Outport  Port=2
  lever23 [m] : Outport  Port=3
  wires:
  Gain5/1 -> offset correction term/1
  Gain3/1 -> length change term/1, variable lever term/1
  Demux/1 -> Gain4/1
  Demux/2 -> lever23 [m]/1
  Gain1/1 -> Demux/1
  Mux/1 -> Gain1/1
  variable lever term/1 -> Mux/2
  Sum1/1 -> Mux/1
  offset correction term/1 -> Sum1/1
  length change term/1 -> Sum1/2
  Constant2/1 -> Sum2/1
  Sum2/1 -> Gain5/1
  Constant1/1 -> Sum2/2, Sum3/1
  Sum3/1 -> Gain3/1
  phi23 [rad]/1 -> Sum3/2
  Product/1 -> Gain2/1
  Constant3/1 -> lever34 [m]/1, Product/2
  Sum4/1 -> Product/1
  Constant5/1 -> Sum4/2
  phi34 [rad]/1 -> Sum4/1
  Gain2/1 -> Sum5/1
  Gain4/1 -> Sum5/3
  Constant4/1 -> Sum5/2
  Sum5/1 -> lmtu [m]/1
